simulink library "Boost_rectifier_average_model_lib_2011"  (Simulink 7.8)
settings: Solver=ode45  StartTime=0.0  StopTime=10.0  RelTol=1e-3
values from neighbouring files (symbols this model uses):
  C = IacRMS*18e-6    [BES_init.m]
  f = 60    [global_parameters.m]
  L = Vdc_nom/(IacRMS*0.2/(2/fs))    [BES_init.m]
  Roff = 1e7    (= 10000000)    [BES_init.m]
  Tds = Ts    (= 8e-05)    [global_parameters.m]
undefined symbols (not defined in the file or in its folder): Vdc_nom
libraries: simulink x1
settings Model: Creator=CH24070  LastModifiedBy=CH24070

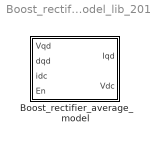
== system Boost_rectifier_average_model_lib_2011 ==
  Boost_rectifier_average_model : Subsystem  mask{C=C, L=L, Roff=Roff, Vdc_nom=Vdc_nom}
      mask prompts: C "DC Bus Capacitance"; L "Boost Inductor"; Roff "Switch resistance when off"; Vdc_nom "Nominal DC Bus Voltage"
      mask init:
      | global_parameters

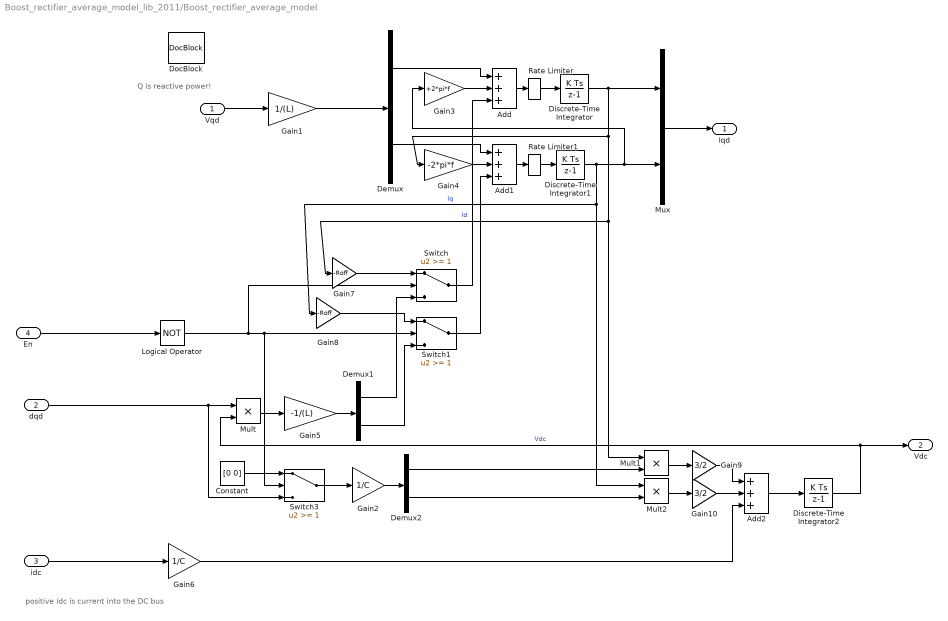
== system Boost_rectifier_average_model_lib_2011/Boost_rectifier_average_model ==
  note: Q is reactive power!
  note: positive idc is current into the DC bus
  Vqd : Inport
  dqd : Inport  Port=2  PortDimensions=2
  idc : Inport  Port=3
  En : Inport  Port=4  OutDataTypeStr=boolean
  Add : Sum  Inputs=+++
  Add1 : Sum  Inputs=+++
  Add2 : Sum  Inputs=+++
  Constant : Constant  Value=[0 0]
  Demux : Demux  Outputs=2
  Demux1 : Demux  Outputs=2
  Demux2 : Demux  Outputs=2
  Discrete-Time Integrator : DiscreteIntegrator  InitialConditionMode=State only (most efficient)  SampleTime=Tds
  Discrete-Time Integrator1 : DiscreteIntegrator  InitialConditionMode=State only (most efficient)  SampleTime=Tds
  Discrete-Time Integrator2 : DiscreteIntegrator  InitialCondition=Vdc_nom  InitialConditionMode=State only (most efficient)  SampleTime=Tds
  DocBlock : simulink/Model-Wide Utilities/DocBlock  DocumentType=Text
  Gain1 : Gain  Gain=1/(L)
  Gain10 : Gain  Gain=3/2
  Gain2 : Gain  Gain=1/C
  Gain3 : Gain  Gain=+2*pi*f
  Gain4 : Gain  Gain=-2*pi*f
  Gain5 : Gain  Gain=-1/(L)
  Gain6 : Gain  Gain=1/C
  Gain7 : Gain  Gain=-Roff
  Gain8 : Gain  Gain=-Roff
  Gain9 : Gain  Gain=3/2
  Logical Operator : Logic  Operator=NOT  AllPortsSameDT=off  OutDataTypeStr=boolean
  Mult : Product  Inputs=**
  Mult1 : Product  Inputs=**
  Mult2 : Product  Inputs=**
  Mux : Mux  Inputs=2
  Rate Limiter : RateLimiter  RisingSlewLimit=1e6  FallingSlewLimit=-1e6  SampleTimeMode=inherited
  Rate Limiter1 : RateLimiter  RisingSlewLimit=1e6  FallingSlewLimit=-1e6  SampleTimeMode=inherited
  Switch : Switch  Threshold=1
  Switch1 : Switch  Threshold=1
  Switch3 : Switch  Threshold=1
  Iqd : Outport
  Vdc : Outport  Port=2
  wires:
  Rate Limiter1/1 -> Discrete-Time Integrator1/1
  Rate Limiter/1 -> Discrete-Time Integrator/1
  Add1/1 -> Rate Limiter1/1
  dqd/1 -> Mult/1, Switch3/3
  Gain8/1 -> Switch1/1
  Discrete-Time Integrator1/1 -> Mux/2, Gain3/1, Mult2/1, Gain8/1  "Iq"
  Demux1/2 -> Switch1/3
  Mult1/1 -> Gain9/1
  Switch1/1 -> Add1/3
  Add/1 -> Rate Limiter/1
  Switch/1 -> Add/3
  Gain1/1 -> Demux/1
  Gain5/1 -> Demux1/1
  Mult2/1 -> Gain10/1
  Constant/1 -> Switch3/1
  Gain9/1 -> Add2/1
  Demux2/2 -> Mult2/2
  idc/1 -> Gain6/1
  Mult/1 -> Gain5/1
  Add2/1 -> Discrete-Time Integrator2/1
  Gain7/1 -> Switch/1
  Demux/1 -> Add/1
  En/1 -> Logical Operator/1
  Discrete-Time Integrator/1 -> Mux/1, Gain4/1, Mult1/1, Gain7/1  "Id"
  Mux/1 -> Iqd/1
  Switch3/1 -> Gain2/1
  Logical Operator/1 -> Switch/2, Switch1/2, Switch3/2
  Gain10/1 -> Add2/2
  Gain6/1 -> Add2/3
  Gain2/1 -> Demux2/1
  Demux1/1 -> Switch/3
  Vqd/1 -> Gain1/1
  Gain4/1 -> Add1/2
  Gain3/1 -> Add/2
  Demux2/1 -> Mult1/2
  Demux/2 -> Add1/1
  Discrete-Time Integrator2/1 -> Vdc/1, Mult/2  "Vdc"
